simulink model "Microgrid"  (R2025a)
settings: Solver=ode23tb  StartTime=0  StopTime=3600  FixedStep=3600  MaxStep=60  MinStep=1e-06  RelTol=0.0001  AbsTol=1e-07
undefined symbols (not defined in the file): Pnom
libraries: simulink x8, spsThreePhaseDynamicLoadLib x3, fuzblock x2, spsThreePhaseSeriesRLCLoadLib x1, rllib x1, spsThreePhaseTransformerTwoWindingsLib x1, spsThreePhaseVIMeasurementLib x1, spsThreePhaseBreakerLib x1, spsThreePhaseSourceLib x1, spspowerguiLib x1
settings Model: Creator=jlesage  LastModifiedBy=86138
settings SolverCC: InitialStep=0.1  ConsecutiveZCsStepRelTol=1000  AlgebraicLoopSolver=TrustRegion
settings DataIOCC: ReturnWorkspaceOutputs=off
settings DebuggingCC: ArithmeticOperatorsInVariantConditions=warning
settings ModelReferenceCC: EnableRefExpFcnMdlSchedulingChecks=on
settings SFSimCC: SimUseLocalCustomCode=off  CustomCodeUndefinedFunction=UseInterfaceOnly
settings RTWCC: RTWUseLocalCustomCode=off  GPUComputeCapability=3.5

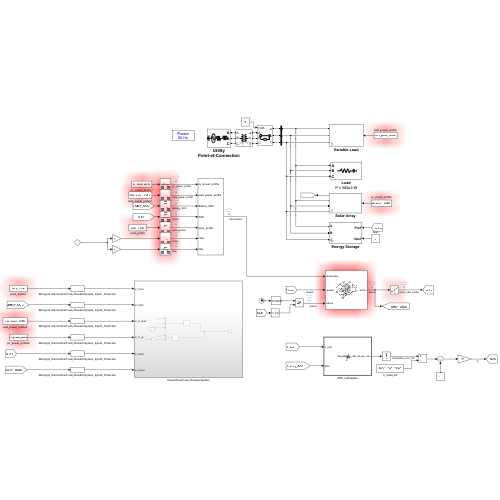
[thumbnail: Simulink's stored preview of the top-level diagram]
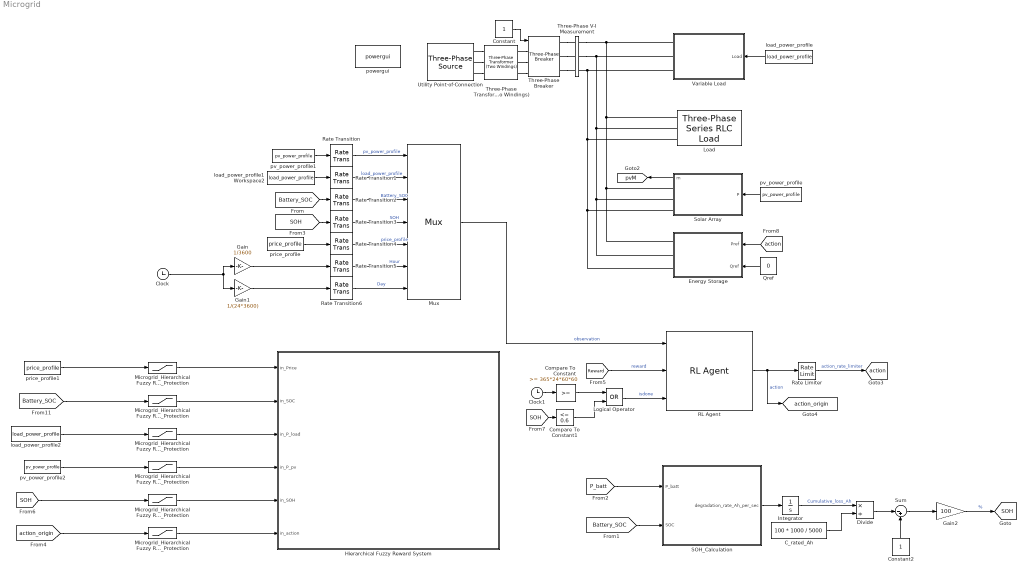
== system Microgrid ==
  C_rated_Ah : Constant  Value=100 * 1000 / 5000
  Clock : Clock
  Clock1 : Clock
  Compare To Constant : simulink/Logic and Bit Operations/Compare To Constant  relop=>=  const=365*24*60*60  OutDataTypeStr=boolean
  Compare To Constant1 : simulink/Logic and Bit Operations/Compare To Constant  relop=<=  const=0.6  OutDataTypeStr=boolean
  Constant : Constant
  Constant2 : Constant
  Divide : Product  Inputs=*/
  Energy Storage : Subsystem  mask(Grid-connected Energy Storage (PQ Model)){Vn=5000, Fn=60, PnomkW=500, kWh_Rated=100, Efficiency=96, LimitVec=[90 10], RechargeSOC=11, Precharge=50, autoRecharge=off, Initial_kWh_pc=80, PQvec=[500e3 0]}
      mask prompts: Vn "Nominal L-L Voltage [Vrms]"; Fn "Nominal Frequency [Hz]"; PnomkW "Rated Power [kW]"; kWh_Rated "Rated Capacity [kWh]"; Efficiency "Overall System Efficiency [%]"; LimitVec "Upper/Lower Charge Limits [%]"; RechargeSOC "SOC to Recharge [%]"; Precharge "Recharge Rate [% of Rated Power]"; autoRecharge "Enable Auto-Recharge"; Initial_kWh_pc "Initial State-of-Charge [0-100%]"; PQvec "Initial Active/Reactive Cmds"
      mask help:
      | The energy storage block models a generic grid-connected energy storage system (ESS), most commonly a battery system. This is a system-level model that does not contain any power electronics, but is useful for load flow, phasor, and hybrid phasor-EMT simulations. The inputs to this block are the commanded active and reactive power of the ESS. The ESS is assumed to have four quadrent operation.
      |
      | For more detailed ESS models, consider the battery block in the Drives library. Consider using this PQ Model to perform load flow studies and switch to a more detailed model when full EMT studies or more advanced controls are required.
      |
      | Note: The initial active/reactive power commands must be specified for use for Load Flow analysis.
      mask init:
      | % Calculate Initial Conditions
      | Pnom = PnomkW*1e3;
      | P0 = -PQvec(1);  Q0 = -PQvec(2);
      | if abs(P0) > Pnom
      |     P0 = sign(P0)*Pnom;
      | end
      | 
      | % Calculate Q0 given Reactive Power Capability Curve
      | Qlim = sqrt(Pnom^2 - P0^2);
      | if Qlim > abs(Q0)
      |     Q0 = sign(Q0)*Qlim;
      | end
      | 
      | UpChrgLim = LimitVec(1);
      | LowChrgLim = LimitVec(2);
      | if Initial_kWh_pc > UpChrgLim && P0 < 0
      |     P0 = 0; Q0 = 0;
      | elseif Initial_kWh_pc < LowChrgLim && P0 > 0
      |     P0 = 0; Q0 = 0;
      | end
      mask DialogControl Container7 Prompt: Grid Connection Properties
      mask DialogControl Container11 Prompt: Charge/Discharge Controls
      mask DialogControl Container12 Prompt: Initial Conditions
  Gain : Gain  Gain=1/3600
  Gain1 : Gain  Gain=1/(24*3600)
  Gain2 : Gain  Gain=100
  Hierarchical Fuzzy Reward System : Subsystem
  Integrator : Integrator
  Load : spsThreePhaseSeriesRLCLoadLib/Three-Phase Series RLC Load  LConnTagsString=A|B|C  Configuration=Y (grounded)  NominalVoltage=5000  Vabc=[1e3 1e3 1e3]  Vabcp=[1e3 1e3 1e3]  NominalFrequency=60  UnbalancedPower=off  ActivePower=500e3  InductivePower=0  CapacitivePower=0  Pabc=[10e3 9e3 11e3]  QLabc=[100 90 110]  QCabc=[100 90 110]  Pabcp=[10e3 9e3 11e3]  QLabcp=[100 90 110]  QCabcp=[100 90 110]  Measurements=None  LoadType=constant Z
      settings: AttributesFormatString=P = %<ActivePower> W
  Logical Operator : Logic  Operator=OR  AllPortsSameDT=off  OutDataTypeStr=boolean
  Microgrid_Hierarchical Fuzzy Reward System_Input1_Protection : Saturate  UpperLimit=2  LowerLimit=0
  Microgrid_Hierarchical Fuzzy Reward System_Input2_Protection : Saturate  UpperLimit=100  LowerLimit=0
  Microgrid_Hierarchical Fuzzy Reward System_Input3_Protection : Saturate  UpperLimit=700000  LowerLimit=-700000
  Microgrid_Hierarchical Fuzzy Reward System_Input4_Protection : Saturate  UpperLimit=10  LowerLimit=-10
  Microgrid_Hierarchical Fuzzy Reward System_Input5_Protection : Saturate  UpperLimit=10  LowerLimit=-10
  Microgrid_Hierarchical Fuzzy Reward System_Input6_Protection : Saturate  UpperLimit=10  LowerLimit=-10
  Mux : Mux  Inputs=7
      settings: DisplayOption=signals
  Qref : Constant  Value=0
  RL Agent : rllib/RL Agent  Agent=agentObj  ExternalActionAsInput=off  ProvideLastAction=off  ProvideCumRwd=off  TreatAsDirectFeedthrough=off  UseStrictObservationDataTypes=on
  Rate Limiter : RateLimiter  RisingSlewLimit=Pnom  FallingSlewLimit=-Pnom  SampleTimeMode=inherited
  Rate Transition{,1..6} (7 alike) : RateTransition  OutPortSampleTime=Ts
  SOH_Calculation : MATLAB Function  TreatAsAtomicUnit=on
  Solar Array : Subsystem  mask(Grid-Connected PV Array (PQ Model)){Vn=5000, Fn=60, P0=500e3}
      mask prompts: Vn "Nominal L-L Voltage [Vrms]"; Fn "Nominal Frequency [Hz]"; P0 "Initial Power [W]"
      mask help:
      | This block models a grid-connected solar array using the Three-Phase Dynamic Load block. This is a system-level model that does not contain any power electronics, but is useful for load flow, phasor, and hybrid phasor-EMT simulations. The input to this block is the power output of the grid connected PV array, not irradiance.
      |
      | For more detailed PV models, consider the PV Array block in the Renewables library. Consider using this PQ Model to perform load flow studies and switch to a more detailed model when full EMT studies are required.
      |
      | Note: The array power must be specified for use for Load Flow analysis.
      mask init:
      | % P0 = Irr0*TotalArea*Efficiency/100;
      | P0 = -P0;
      mask Display:
      | color('white')
      | port_label('input',1,'P')
      | port_label('output',1,'m')
      | port_label('Rconn',1,'A')
      | port_label('Rconn',2,'B')
      | port_label('Rconn',3,'C')
  Sum : Sum  Inputs=|-+
  Three-Phase Transformer (Two Windings) : spsThreePhaseTransformerTwoWindingsLib/Three-Phase Transformer (Two Windings)  Winding1Connection=Yg  Winding2Connection=Yg  CoreType=Three single-phase transformers  SetSaturation=off  Hysteresis=off  DataFile='hysteresis'  SetInitialFlux=off  Measurements=None  UNITS=pu  NominalPower=[ 250e6 , 60 ]  Winding1=[ 13.8e3 , 0.002 , 0.08 ]  Winding2=[ 5000 , 0.002 , 0.08 ]  Rm=500  Lm=500  L0=0.5  Saturation=[ 0,0 ; 0.0024,1.2 ; 1.0,1.52 ]  InitialFluxes=[ 0.8 , -0.8 , 0.7 ]  BreakLoop=off  DiscreteSolver=Trapezoidal iterative  DataType=off  TransfoNumber=1
  Three-Phase V-I Measurement : spsThreePhaseVIMeasurementLib/Three-Phase V-I Measurement  VoltageMeasurement=phase-to-ground  SetLabelV=on  LabelV=Vabc  Vpu=off  VpuLL=off  CurrentMeasurement=yes  SetLabelI=on  LabelI=Iabc  Ipu=off  Pbase=100e6  Vbase=500e3  OutputType=Complex  PhasorSimulation=on  PSBequivalent=0
  Three-Phase Breaker : spsThreePhaseBreakerLib/Three-Phase Breaker  InitialState=closed  SwitchA=on  SwitchB=on  SwitchC=on  SwitchTimes="[1/60  5/60]"  External=on  BreakerResistance=0.01  SnubberResistance=1e6  SnubberCapacitance=inf  Measurements=None
  Utility Point-of-Connection : spsThreePhaseSourceLib/Three-Phase Source  InternalConnection=Yg  VoltagePhases=off  Voltage=(13800)*1.00243  PhaseAngle=0.071468  Voltage_phases=[25e3 25e3 25e3]/sqrt(3)  PhaseAngles_phases=[0 -120 +120]  Frequency=60  NonIdealSource=on  SpecifyImpedance=on  Resistance=0.8929  Inductance=16.58e-3  ShortCircuitLevel=250e6  BaseVoltage=13.8e3  XRratio=7  BusType=swing  Pref=10e3  Qref=0  Prefabc=[10e3, 10e3, 10e3]  Qrefabc=[0, 0, 0]  Qmin=-inf  Qmax=inf
  Variable Load : Subsystem  mask(Variable Load (PQ Model)){Vn=5000, Fn=60, PF=1, Load0=200e3}
      mask prompts: Vn "Nominal L-L Voltage [Vrms]"; Fn "Nominal Frequency [Hz]"; PF "Power Factor [0 to 1]"; Load0 "Initial Load [W]"
      mask help:
      | The Variable Load block is a lumped approximation for a distribution feeder. For non-unity power factor loads, the input (active power) is scaled accordingly to generate a desired load.
      |
      | Note: The initial input load must be specified for use for Load Flow analysis.
      mask init:
      | P0 = Load0;
      | Q0 = Load0*sqrt(1/PF-1);
      mask Display:
      | color('white')
      | port_label('input',1,'Load')
      | port_label('Rconn',1,'A')
      | port_label('Rconn',2,'B')
      | port_label('Rconn',3,'C')
  load_power_profile : FromWorkspace  VariableName=load_power_profile  SampleTime=3600
  load_power_profile1 Workspace2 : FromWorkspace  VariableName=load_power_profile  SampleTime=3600
  load_power_profile2 : FromWorkspace  VariableName=load_power_profile  SampleTime=3600
  powergui : spspowerguiLib/powergui  Priority=1  SimulationMode=Phasor  SampleTime=1e-4  frequency=60  Iterations=50  frequencyindice=60  Pbase=100e6  ErrMax=0.0001  UnitsV=kV  UnitsW=MW  buscounter=3  FunctionMessages=off  echomessages=off  EnableUseOfTLC=off  CurrentSourceSwitches=off  DisableSnubberDevices=off  DisableRonSwitches=off  DisableVfSwitches=off  DisplayEquations=off  AutomaticDiscreteSolvers=off  SolverType=Tustin/Backward Euler (TBE)  Interpol=off  ExternalGateDelay=off  methode=off  Ts=100  x0status=blocks  SPID=on  SwTol=0  HookPort=off  NonlinearTolerance=1e-4  nMaxIteration=100  ContinueOnMaxIteration=off  RestoreLinks=warning  ResistiveCurrentMeasurement=off  Frange=[0:2:500]  Ylog=off  Xlog=on  ShowGrid=off  save=off  variable=ZData  structure=0  ZoomFFT=off  StartTime=0.0  cycles=1  DisplayStyle=1  fundamental=60  FreqAxis=off  MaxFrequency=1000  frequencyindicesteady=1  RmsSteady=1  display=off
  price_profile : FromWorkspace  VariableName=price_profile  SampleTime=3600
  price_profile1 : FromWorkspace  VariableName=price_profile  SampleTime=3600
  pv_power_profile : FromWorkspace  VariableName=pv_power_profile  SampleTime=3600
  pv_power_profile1 : FromWorkspace  VariableName=pv_power_profile  SampleTime=3600
  pv_power_profile2 : FromWorkspace  VariableName=pv_power_profile  SampleTime=3600
  tag scope: SOH=global, action=global, action_origin=global, pvM=global
  wires:
  Constant/1 -> Three-Phase Breaker/1
  pv_power_profile/1 -> Solar Array/1(P)
  load_power_profile/1 -> Variable Load/1(Load)
  Solar Array/1(m) -> [pvM]
  Mux/1 -> RL Agent/1  "observation"
  pv_power_profile1/1 -> Rate Transition/1
  load_power_profile1 Workspace2/1 -> Rate Transition1/1
  [Battery_SOC] -> Rate Transition2/1
  price_profile/1 -> Rate Transition4/1
  Gain/1 -> Rate Transition5/1
  Gain1/1 -> Rate Transition6/1
  Clock/1 -> Gain1/1, Gain/1
  Qref/1 -> Energy Storage/2(Qref)
  [Battery_SOC] -> SOH_Calculation/2(SOC)
  [P_batt] -> SOH_Calculation/1(P_batt)
  SOH_Calculation/1(degradation_rate_Ah_per_sec) -> Integrator/1
  Integrator/1 -> Divide/1  "Cumulative_loss_Ah"
  C_rated_Ah/1 -> Divide/2
  Divide/1 -> Sum/1
  Constant2/1 -> Sum/2
  Sum/1 -> Gain2/1
  [SOH] -> Rate Transition3/1
  [Reward] -> RL Agent/2  "reward"
  Logical Operator/1 -> RL Agent/3  "isdone"
  Clock1/1 -> Compare To Constant/1
  Compare To Constant/1 -> Logical Operator/1
  [SOH] -> Compare To Constant1/1
  Compare To Constant1/1 -> Logical Operator/2
  [action] -> Energy Storage/1(Pref)
  RL Agent/1 -> [action_origin], Rate Limiter/1  "action"
  Rate Transition/1 -> Mux/1  "pv_power_profile"
  Rate Transition1/1 -> Mux/2  "load_power_profile"
  Rate Transition2/1 -> Mux/3  "Battery_SOC"
  Rate Transition3/1 -> Mux/4  "SOH"
  Rate Transition4/1 -> Mux/5  "price_profile"
  Rate Transition5/1 -> Mux/6  "Hour"
  Rate Transition6/1 -> Mux/7  "Day"
  Rate Limiter/1 -> [action]  "action_rate_limiter"
  price_profile1/1 -> Microgrid_Hierarchical Fuzzy Reward System_Input1_Protection/1
  Microgrid_Hierarchical Fuzzy Reward System_Input1_Protection/1 -> Hierarchical Fuzzy Reward System/1(in_Price)
  [Battery_SOC] -> Microgrid_Hierarchical Fuzzy Reward System_Input2_Protection/1
  Microgrid_Hierarchical Fuzzy Reward System_Input2_Protection/1 -> Hierarchical Fuzzy Reward System/2(in_SOC)
  load_power_profile2/1 -> Microgrid_Hierarchical Fuzzy Reward System_Input3_Protection/1
  Microgrid_Hierarchical Fuzzy Reward System_Input3_Protection/1 -> Hierarchical Fuzzy Reward System/3(in_P_load)
  pv_power_profile2/1 -> Microgrid_Hierarchical Fuzzy Reward System_Input4_Protection/1
  Microgrid_Hierarchical Fuzzy Reward System_Input4_Protection/1 -> Hierarchical Fuzzy Reward System/4(in_P_pv)
  [SOH] -> Microgrid_Hierarchical Fuzzy Reward System_Input5_Protection/1
  Microgrid_Hierarchical Fuzzy Reward System_Input5_Protection/1 -> Hierarchical Fuzzy Reward System/5(in_SOH)
  [action_origin] -> Microgrid_Hierarchical Fuzzy Reward System_Input6_Protection/1
  Microgrid_Hierarchical Fuzzy Reward System_Input6_Protection/1 -> Hierarchical Fuzzy Reward System/6(in_action)
  Gain2/1 -> [SOH]  "%"
  connections:
  Utility Point-of-Connection/RConn1 -- Three-Phase Transformer (Two Windings)/LConn1
  Utility Point-of-Connection/RConn2 -- Three-Phase Transformer (Two Windings)/LConn2
  Utility Point-of-Connection/RConn3 -- Three-Phase Transformer (Two Windings)/LConn3
  Three-Phase Transformer (Two Windings)/RConn1 -- Three-Phase Breaker/LConn1
  Three-Phase Transformer (Two Windings)/RConn2 -- Three-Phase Breaker/LConn2
  Three-Phase Transformer (Two Windings)/RConn3 -- Three-Phase Breaker/LConn3
  Load/LConn1 -- Variable Load/RConn1 -- Three-Phase V-I Measurement/RConn1 -- Solar Array/RConn1 -- Energy Storage/RConn1
  Load/LConn2 -- Three-Phase V-I Measurement/RConn2 -- Variable Load/RConn2 -- Energy Storage/RConn2 -- Solar Array/RConn2
  Load/LConn3 -- Three-Phase V-I Measurement/RConn3 -- Variable Load/RConn3 -- Energy Storage/RConn3 -- Solar Array/RConn3
  Three-Phase Breaker/RConn1 -- Three-Phase V-I Measurement/LConn1
  Three-Phase Breaker/RConn2 -- Three-Phase V-I Measurement/LConn2
  Three-Phase Breaker/RConn3 -- Three-Phase V-I Measurement/LConn3

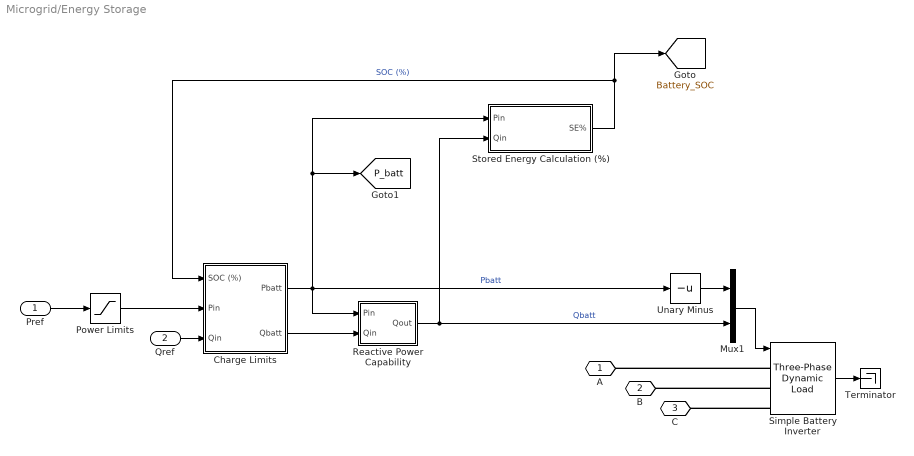
== system Microgrid/Energy Storage ==
  Pref : Inport
  Qref : Inport  Port=2
  Charge Limits : Subsystem
  Mux1 : Mux  Inputs=2
  Power Limits : Saturate  UpperLimit=Pnom  LowerLimit=-Pnom
  Reactive Power Capability : Subsystem
  Simple Battery Inverter : spsThreePhaseDynamicLoadLib/Three-Phase Dynamic Load  NominalVoltage=[Vn Fn]  ActiveReactivePowers=[-500000 -3.38813e-13]  PositiveSequence=[0.999844 -0.0038635]  ExternalControl=on  NpNq=[1.3 2]  TimeConstants="[0  0  0  0]"  MinimumVoltage=0.7  Tfilter=1e-2  LoadFlowParameters=[4,0,0,0,0]
      settings: LibrarySourceBlock=|
      | sps_lib/Passives/Three-Phase
      | Dynamic Load
  Stored Energy Calculation (%) : Subsystem
  Terminator : Terminator
  Unary Minus : UnaryMinus
  A : PMIOPort  Side=Right
  B : PMIOPort  Port=2  Side=Right
  C : PMIOPort  Port=3  Side=Right
  tag scope: Battery_SOC=global, P_batt=global
  wires:
  Charge Limits/2(Qbatt) -> Reactive Power Capability/2(Qin)
  Qref/1 -> Charge Limits/3(Qin)
  Power Limits/1 -> Charge Limits/2(Pin)
  Charge Limits/1(Pbatt) -> Reactive Power Capability/1(Pin), Unary Minus/1, [P_batt], Stored Energy Calculation (%)/1(Pin)  "Pbatt"
  Stored Energy Calculation (%)/1(SE%) -> [Battery_SOC], Charge Limits/1(SOC (%))  "SOC (%)"
  Pref/1 -> Power Limits/1
  Reactive Power Capability/1(Qout) -> Mux1/2, Stored Energy Calculation (%)/2(Qin)  "Qbatt"
  Simple Battery Inverter/1 -> Terminator/1
  Mux1/1 -> Simple Battery Inverter/1
  Unary Minus/1 -> Mux1/1
  connections:
  Simple Battery Inverter/LConn1 -- A/RConn1
  Simple Battery Inverter/LConn3 -- C/RConn1
  Simple Battery Inverter/LConn2 -- B/RConn1

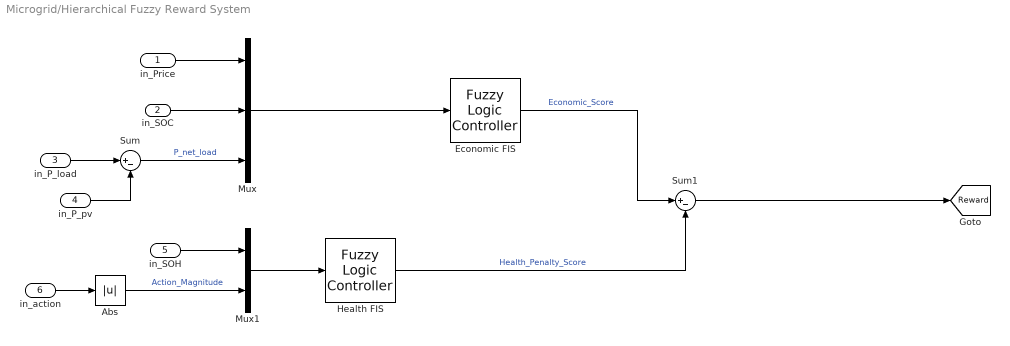
== system Microgrid/Hierarchical Fuzzy Reward System ==
  in_Price : Inport
  in_SOC : Inport  Port=2
  in_P_load : Inport  Port=3
  in_P_pv : Inport  Port=4
  in_SOH : Inport  Port=5
  in_action : Inport  Port=6
  Abs : Abs  SaturateOnIntegerOverflow=off
  Economic FIS : fuzblock/Fuzzy Logic  Controller  FIS='Economic_Reward_FIS.fis'  OutputSampleNumber=101  DataType=double  UseLookupTable=off  NumBreakpoints=10  FuzzifiedInputs=off  RuleFiringStrengths=off  RuleOutputs=off  AggregatedOutputs=off  SimulateUsing=Interpreted execution  OutOfRangeInputValueMessage=warning  NoRuleFiredMessage=warning  EmptyOutputFuzzySetMessage=warning
  Health FIS : fuzblock/Fuzzy Logic  Controller  FIS='Health_Penalty_FIS'  OutputSampleNumber=101  DataType=double  UseLookupTable=off  NumBreakpoints=10  FuzzifiedInputs=off  RuleFiringStrengths=off  RuleOutputs=off  AggregatedOutputs=off  SimulateUsing=Interpreted execution  OutOfRangeInputValueMessage=warning  NoRuleFiredMessage=warning  EmptyOutputFuzzySetMessage=warning
  Mux : Mux  Inputs=3
  Mux1 : Mux  Inputs=2
  Sum : Sum  Inputs=|+-
  Sum1 : Sum  Inputs=|+-
  tag scope: Reward=global
  wires:
  in_P_load/1 -> Sum/1
  in_P_pv/1 -> Sum/2
  Sum/1 -> Mux/3  "P_net_load"
  in_action/1 -> Abs/1
  Abs/1 -> Mux1/2  "Action_Magnitude"
  in_SOH/1 -> Mux1/1
  in_Price/1 -> Mux/1
  in_SOC/1 -> Mux/2
  Economic FIS/1 -> Sum1/1  "Economic_Score"
  Health FIS/1 -> Sum1/2  "Health_Penalty_Score"
  Sum1/1 -> [Reward]
  Mux/1 -> Economic FIS/1
  Mux1/1 -> Health FIS/1

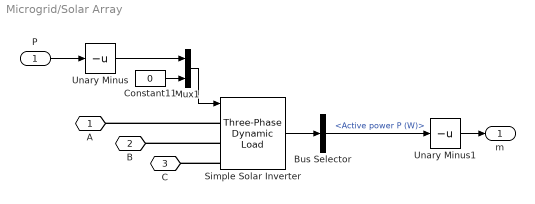
== system Microgrid/Solar Array ==
  P : Inport
  Bus Selector : BusSelector  OutputSignals=Active power P (W)
  Constant11 : Constant  Value=0
  Mux1 : Mux  Inputs=2
  Simple Solar Inverter : spsThreePhaseDynamicLoadLib/Three-Phase Dynamic Load  NominalVoltage=[Vn Fn]  ActiveReactivePowers=[-250000 -3.38813e-13]  PositiveSequence=[0.999844 -0.0038635]  ExternalControl=on  NpNq=[1.3 2]  TimeConstants="[0  0  0  0]"  MinimumVoltage=0.7  Tfilter=1e-2  LoadFlowParameters=[4,0,0,0,0]
      settings: LibrarySourceBlock=|
      | sps_lib/Passives/Three-Phase
      | Dynamic Load
  Unary Minus : UnaryMinus
  Unary Minus1 : UnaryMinus
  A : PMIOPort  Side=Right
  B : PMIOPort  Port=2  Side=Right
  C : PMIOPort  Port=3  Side=Right
  m : Outport  VectorParamsAs1DForOutWhenUnconnected=off
  wires:
  P/1 -> Unary Minus/1
  Unary Minus/1 -> Mux1/1
  Mux1/1 -> Simple Solar Inverter/1
  Constant11/1 -> Mux1/2
  Simple Solar Inverter/1 -> Bus Selector/1
  Bus Selector/1 -> Unary Minus1/1  "<Active power P (W)>"
  Unary Minus1/1 -> m/1
  connections:
  Simple Solar Inverter/LConn2 -- B/RConn1
  Simple Solar Inverter/LConn3 -- C/RConn1
  Simple Solar Inverter/LConn1 -- A/RConn1

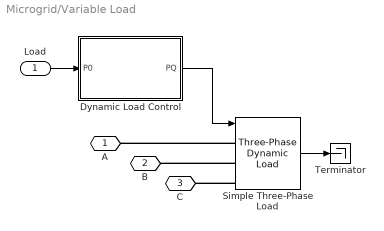
== system Microgrid/Variable Load ==
  Load : Inport
  Dynamic Load Control : Subsystem
  Simple Three-Phase Load : spsThreePhaseDynamicLoadLib/Three-Phase Dynamic Load  NominalVoltage=[Vn Fn]  ActiveReactivePowers=[200000 45883.1]  PositiveSequence=[0.999844 -0.0038635]  ExternalControl=on  NpNq=[1.3 2]  TimeConstants="[0  0  0  0]"  MinimumVoltage=0.7  Tfilter=1e-2  LoadFlowParameters=[4,0,0,0,0]
      settings: LibrarySourceBlock=|
      | sps_lib/Passives/Three-Phase
      | Dynamic Load
  Terminator : Terminator
  A : PMIOPort  Side=Right
  B : PMIOPort  Port=2  Side=Right
  C : PMIOPort  Port=3  Side=Right
  wires:
  Simple Three-Phase Load/1 -> Terminator/1
  Load/1 -> Dynamic Load Control/1(P0)
  Dynamic Load Control/1(PQ) -> Simple Three-Phase Load/1
  connections:
  Simple Three-Phase Load/LConn1 -- A/RConn1
  Simple Three-Phase Load/LConn3 -- C/RConn1
  Simple Three-Phase Load/LConn2 -- B/RConn1

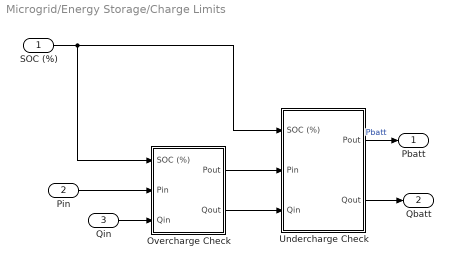
== system Microgrid/Energy Storage/Charge Limits ==
  SOC (%) : Inport
  Pin : Inport  Port=2
  Qin : Inport  Port=3
  Overcharge Check : Subsystem
  Undercharge Check : Subsystem
  Pbatt : Outport  VectorParamsAs1DForOutWhenUnconnected=off
  Qbatt : Outport  Port=2  VectorParamsAs1DForOutWhenUnconnected=off
  wires:
  SOC (%)/1 -> Overcharge Check/1(SOC (%)), Undercharge Check/1(SOC (%))
  Undercharge Check/2(Qout) -> Qbatt/1
  Pin/1 -> Overcharge Check/2(Pin)
  Overcharge Check/1(Pout) -> Undercharge Check/2(Pin)
  Qin/1 -> Overcharge Check/3(Qin)
  Undercharge Check/1(Pout) -> Pbatt/1  "Pbatt"
  Overcharge Check/2(Qout) -> Undercharge Check/3(Qin)

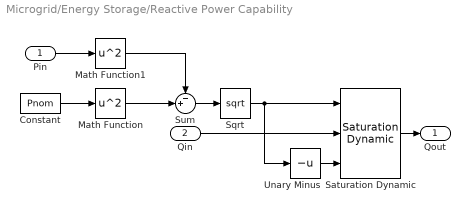
== system Microgrid/Energy Storage/Reactive Power Capability ==
  Pin : Inport
  Qin : Inport  Port=2
  Constant : Constant  Value=Pnom
  Math Function : Math  Operator=square  SignedPower=on
  Math Function1 : Math  Operator=square  SignedPower=on
  Saturation Dynamic : simulink/Discontinuities/Saturation Dynamic  OutMin=[]  OutMax=[]  OutDataTypeStr=Inherit: Same as second input  OutDataType=fixdt(1, 16)  OutScaling=2^-10  DoSatur=off
  Sqrt : Sqrt
  Sum : Sum  Inputs=-+|
  Unary Minus : UnaryMinus
  Qout : Outport  VectorParamsAs1DForOutWhenUnconnected=off
  wires:
  Sqrt/1 -> Saturation Dynamic/1, Unary Minus/1
  Math Function1/1 -> Sum/1
  Math Function/1 -> Sum/2
  Constant/1 -> Math Function/1
  Sum/1 -> Sqrt/1
  Unary Minus/1 -> Saturation Dynamic/3
  Saturation Dynamic/1 -> Qout/1
  Pin/1 -> Math Function1/1
  Qin/1 -> Saturation Dynamic/2

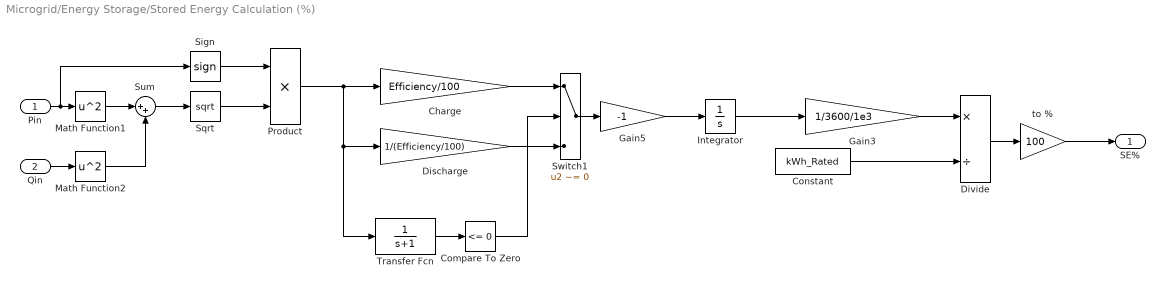
== system Microgrid/Energy Storage/Stored Energy Calculation (%) ==
  Pin : Inport
  Qin : Inport  Port=2
  Charge : Gain  Gain=Efficiency/100
  Compare To Zero : simulink/Logic and Bit Operations/Compare To Zero  relop=<=  OutDataTypeStr=boolean
  Constant : Constant  Value=kWh_Rated
  Discharge : Gain  Gain=1/(Efficiency/100)
  Divide : Product  Inputs=*/
  Gain3 : Gain  Gain=1/3600/1e3
  Gain5 : Gain  Gain=-1
  Integrator : Integrator  InitialCondition=(Initial_kWh_pc/100)*kWh_Rated*3600*1e3  LimitOutput=on  UpperSaturationLimit=kWh_Rated * 3600000  LowerSaturationLimit=0
  Math Function1 : Math  Operator=square  SignedPower=on
  Math Function2 : Math  Operator=square  SignedPower=on
  Product : Product
  Sign : Signum
  Sqrt : Sqrt
  Sum : Sum  Inputs=|++
  Switch1 : Switch  Criteria=u2 ~= 0  SaturateOnIntegerOverflow=off  InputSameDT=off
  Transfer Fcn : TransferFcn  Denominator=[1 1]
  to % : Gain  Gain=100
  SE% : Outport  VectorParamsAs1DForOutWhenUnconnected=off
  wires:
  Sign/1 -> Product/1
  Sqrt/1 -> Product/2
  Sum/1 -> Sqrt/1
  Math Function2/1 -> Sum/2
  Math Function1/1 -> Sum/1
  Qin/1 -> Math Function2/1
  Pin/1 -> Math Function1/1, Sign/1
  Product/1 -> Transfer Fcn/1, Discharge/1, Charge/1
  Discharge/1 -> Switch1/3
  Gain5/1 -> Integrator/1
  to %/1 -> SE%/1
  Transfer Fcn/1 -> Compare To Zero/1
  Switch1/1 -> Gain5/1
  Gain3/1 -> Divide/1
  Charge/1 -> Switch1/1
  Divide/1 -> to %/1
  Compare To Zero/1 -> Switch1/2
  Integrator/1 -> Gain3/1
  Constant/1 -> Divide/2

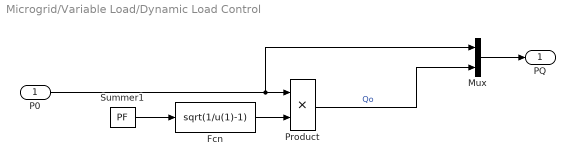
== system Microgrid/Variable Load/Dynamic Load Control ==
  P0 : Inport
  Fcn : Fcn  Expr=sqrt(1/u(1)-1)
  Mux : Mux  Inputs=2
  Product : Product
  Summer1 : Constant  Value=PF
  PQ : Outport  VectorParamsAs1DForOutWhenUnconnected=off
  wires:
  Summer1/1 -> Fcn/1
  Fcn/1 -> Product/2
  P0/1 -> Product/1, Mux/1
  Mux/1 -> PQ/1
  Product/1 -> Mux/2  "Qo"

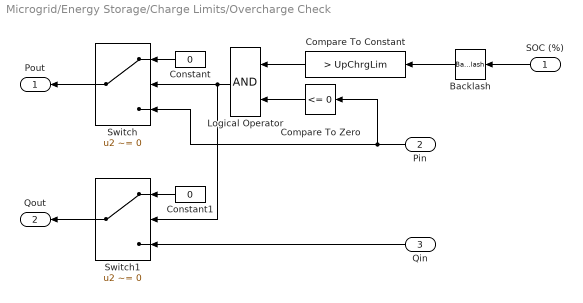
== system Microgrid/Energy Storage/Charge Limits/Overcharge Check ==
  SOC (%) : Inport
  Pin : Inport  Port=2
  Qin : Inport  Port=3
  Backlash : Backlash  BacklashWidth=1e-3  InitialOutput=Initial_kWh_pc  ZeroCross=off
  Compare To Constant : simulink/Logic and Bit Operations/Compare To Constant  relop=>  const=UpChrgLim  OutDataTypeStr=boolean
  Compare To Zero : simulink/Logic and Bit Operations/Compare To Zero  relop=<=  OutDataTypeStr=boolean
  Constant : Constant  Value=0
  Constant1 : Constant  Value=0
  Logical Operator : Logic  AllPortsSameDT=off  OutDataTypeStr=boolean
  Switch : Switch  Criteria=u2 ~= 0  SaturateOnIntegerOverflow=off  InputSameDT=off
  Switch1 : Switch  Criteria=u2 ~= 0  SaturateOnIntegerOverflow=off  InputSameDT=off
  Pout : Outport  VectorParamsAs1DForOutWhenUnconnected=off
  Qout : Outport  Port=2  VectorParamsAs1DForOutWhenUnconnected=off
  wires:
  Backlash/1 -> Compare To Constant/1
  Switch1/1 -> Qout/1
  Constant1/1 -> Switch1/1
  Qin/1 -> Switch1/3
  Compare To Zero/1 -> Logical Operator/2
  Switch/1 -> Pout/1
  Pin/1 -> Switch/3, Compare To Zero/1
  SOC (%)/1 -> Backlash/1
  Constant/1 -> Switch/1
  Logical Operator/1 -> Switch/2, Switch1/2
  Compare To Constant/1 -> Logical Operator/1

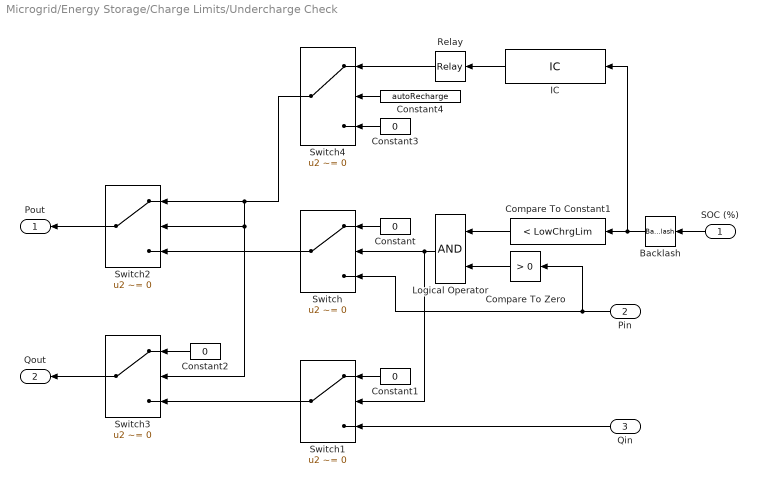
== system Microgrid/Energy Storage/Charge Limits/Undercharge Check ==
  SOC (%) : Inport
  Pin : Inport  Port=2
  Qin : Inport  Port=3
  Backlash : Backlash  BacklashWidth=1e-3  InitialOutput=Initial_kWh_pc  ZeroCross=off
  Compare To Constant1 : simulink/Logic and Bit Operations/Compare To Constant  relop=<  const=LowChrgLim  OutDataTypeStr=boolean
  Compare To Zero : simulink/Logic and Bit Operations/Compare To Zero  relop=>  OutDataTypeStr=boolean
  Constant{,1..3} (4 alike) : Constant  Value=0
  Constant4 : Constant  Value=autoRecharge
  IC : InitialCondition  Value=RechargeSOC
  Logical Operator : Logic  AllPortsSameDT=off  OutDataTypeStr=boolean
  Relay : Relay  OnSwitchValue=RechargeSOC  OffSwitchValue=LowChrgLim  OnOutputValue=0  OffOutputValue=-Precharge/100*Pnom
  Switch{,1..4} (5 alike) : Switch  Criteria=u2 ~= 0  SaturateOnIntegerOverflow=off  InputSameDT=off
  Pout : Outport  VectorParamsAs1DForOutWhenUnconnected=off
  Qout : Outport  Port=2  VectorParamsAs1DForOutWhenUnconnected=off
  wires:
  Constant4/1 -> Switch4/2
  Constant3/1 -> Switch4/3
  Relay/1 -> Switch4/1
  Constant2/1 -> Switch3/1
  Switch1/1 -> Switch3/3
  Switch3/1 -> Qout/1
  Switch2/1 -> Pout/1
  Switch/1 -> Switch2/3
  IC/1 -> Relay/1
  Switch4/1 -> Switch3/2, Switch2/2, Switch2/1
  Backlash/1 -> Compare To Constant1/1, IC/1
  Qin/1 -> Switch1/3
  Constant1/1 -> Switch1/1
  Compare To Constant1/1 -> Logical Operator/1
  Logical Operator/1 -> Switch1/2, Switch/2
  Constant/1 -> Switch/1
  SOC (%)/1 -> Backlash/1
  Pin/1 -> Compare To Zero/1, Switch/3
  Compare To Zero/1 -> Logical Operator/2

== matlab function Microgrid/SOH_Calculation ==
  data: P_batt input; degradation_rate_Ah_per_sec output; SOC input
function degradation_rate_Ah_per_sec = fcn(P_batt, SOC)
% 本函数根据电池功率和SOC，计算瞬时的容量衰减速率（单位：安时/秒）

% --- 1. 从模型Mask传入的参数 (在fcn模块的Ports and Data Manager中定义为Parameter) ---
% 假设这些参数已经通过对话框传入
V_nom_ph = 5000 / sqrt(3); % 标称相电压
C_rated_Ah = 100 * 1000 / 5000; % 初始额定容量 (Ah)

% --- 2. 老化模型参数 (这些是经验值，需要根据具体电池型号或文献来标定) ---
% 循环老化系数
k_delta = 1.4e-5; % DOD对老化的影响因子
k_c = 0.05;       % 充放电倍率对老化的影响因子
% 日历老化系数
k_t = 7.5e-7;     % 日历老化基础速率 (1/sqrt(day))
k_soc = 20;       % SOC对日历老化的影响因子

% --- 3. 计算中间变量 ---
I_batt = P_batt / V_nom_ph;      % 电池电流 (A)
C_rate = abs(I_batt) / C_rated_Ah; % 充放电倍率 (C)

% --- 4. 计算循环老化速率 (Cycle Aging) ---
% DOD的影响，这里用SOC的U型曲线来近似，SOC在0.5附近老化最慢
DOD_stress = 1 + k_delta * ( (SOC/100 - 0.5)^2 ); 
% C-rate的影响
C_rate_stress = 1 + k_c * C_rate;

% 循环老化导致的容量损失速率（单位：Ah/s）
% 正比于电流的绝对值，并受到DOD和C-rate的加剧
cycle_loss_rate = DOD_stress * C_rate_stress * abs(I_batt) * (1e-7);

% --- 5. 计算日历老化速率 (Calendar Aging) ---
% 正比于SOC，SOC越高，静置老化越快
% 转换为秒为单位
calendar_loss_rate_per_day = k_t * exp(k_soc * (SOC/100 - 0.5));
calendar_loss_rate = calendar_loss_rate_per_day * C_rated_Ah / (24*3600);

% --- 6. 计算总老化速率 ---
% 总容量损失速率是两者之和（在某些模型中可能是取较大值）
degradation_rate_Ah_per_sec = cycle_loss_rate + calendar_loss_rate;

end
